simulink model "s47_249_t"  (R2019a)
settings: Solver=VariableStepAuto  StartTime=0.0  StopTime=3800  RelTol=1e-3
settings Model: Creator=Administrator  LastModifiedBy=Administrator

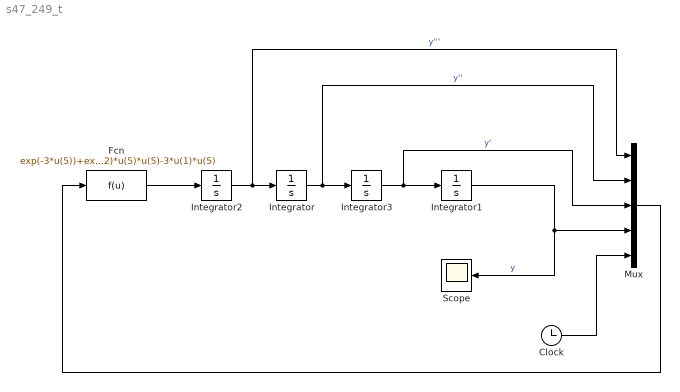
== system s47_249_t ==
  Clock : Clock
  Fcn : Fcn  Expr=exp(-3*u(5))+exp(-5*u(5))*sin(4*u(5)+pi/3)-5*u(4)-4*u(3)-3*u(2)*u(5)*u(5)-3*u(1)*u(5)
  Integrator : Integrator  InitialCondition=0.5
  Integrator1 : Integrator  InitialCondition=1
  Integrator2 : Integrator  InitialCondition=0.2
  Integrator3 : Integrator  InitialCondition=0.5
  Mux : Mux  Inputs=5
  Scope : Scope
  wires:
  Integrator3/1 -> Mux/3, Integrator1/1  "y'"
  Integrator1/1 -> Scope/1, Mux/4  "y"
  Mux/1 -> Fcn/1
  Integrator2/1 -> Mux/1, Integrator/1  "y'''"
  Integrator/1 -> Mux/2, Integrator3/1  "y''"
  Clock/1 -> Mux/5
  Fcn/1 -> Integrator2/1
